simulink model "MechSubTest"  (R2016b)
settings: Solver=VariableStepAuto  StartTime=0.0  StopTime=10.0  RelTol=1e-3
libraries: simulink x1
settings Model: Creator=liana  LastModifiedBy=liana

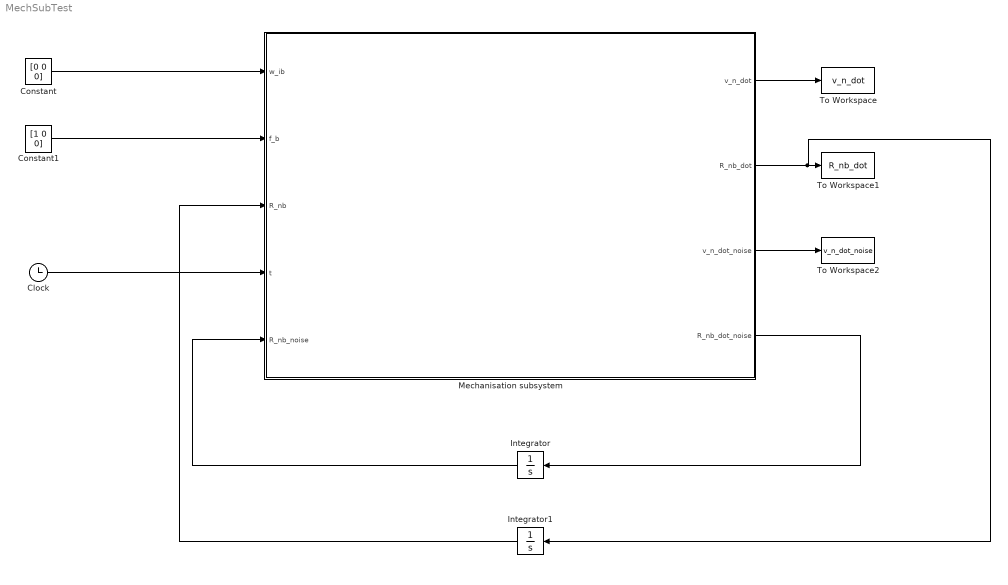
== system MechSubTest ==
  Clock : Clock
  Constant : Constant  Value=[0 0 0]
  Constant1 : Constant  Value=[1 0 0]
  Integrator : Integrator
  Integrator1 : Integrator
  Mechanisation subsystem : Subsystem
  To Workspace : ToWorkspace  VariableName=v_n_dot  SampleTime=-1
  To Workspace1 : ToWorkspace  VariableName=R_nb_dot  SampleTime=-1
  To Workspace2 : ToWorkspace  VariableName=v_n_dot_noise  SampleTime=-1
  wires:
  Constant/1 -> Mechanisation subsystem/1(w_ib)
  Constant1/1 -> Mechanisation subsystem/2(f_b)
  Mechanisation subsystem/2(R_nb_dot) -> Integrator1/1, To Workspace1/1
  Clock/1 -> Mechanisation subsystem/4(t)
  Mechanisation subsystem/4(R_nb_dot_noise) -> Integrator/1
  Integrator/1 -> Mechanisation subsystem/5(R_nb_noise)
  Mechanisation subsystem/1(v_n_dot) -> To Workspace/1
  Mechanisation subsystem/3(v_n_dot_noise) -> To Workspace2/1
  Integrator1/1 -> Mechanisation subsystem/3(R_nb)

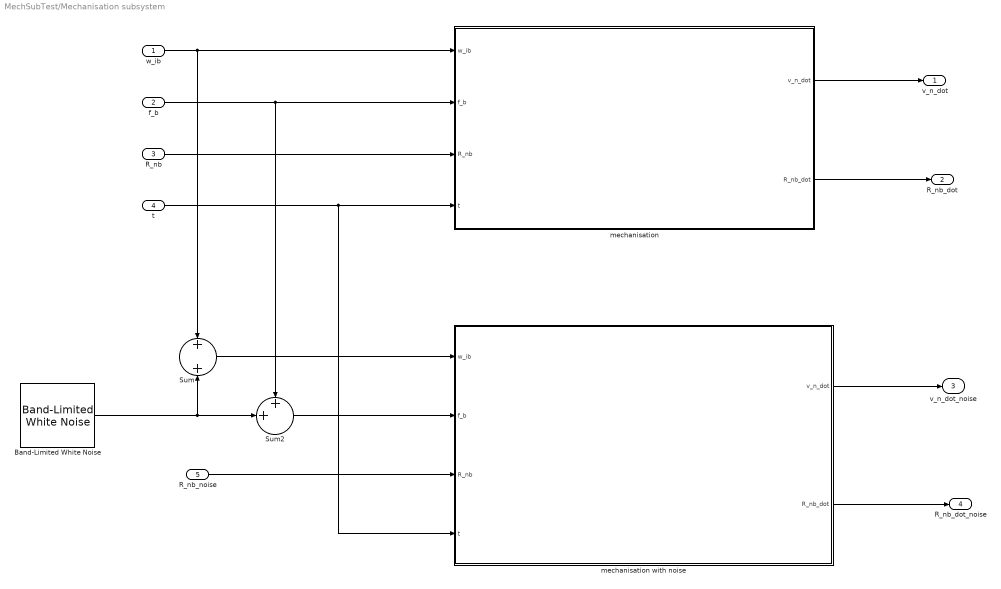
== system MechSubTest/Mechanisation subsystem ==
  w_ib : Inport
  f_b : Inport  Port=2
  R_nb : Inport  Port=3
  t : Inport  Port=4
  R_nb_noise : Inport  Port=5
  Band-Limited White Noise : simulink/Sources/Band-Limited White Noise  Cov=[100 100 100]'  Ts=0.1  seed=[23341]  VectorParams1D=off
  Sum : Sum  Inputs=+|+
  Sum2 : Sum  Inputs=++|
  mechanisation : MATLAB Function  TreatAsAtomicUnit=on
  mechanisation with noise : MATLAB Function  TreatAsAtomicUnit=on
  v_n_dot : Outport
  R_nb_dot : Outport  Port=2
  v_n_dot_noise : Outport  Port=3
  R_nb_dot_noise : Outport  Port=4
  wires:
  w_ib/1 -> mechanisation/1(w_ib), Sum/1
  t/1 -> mechanisation with noise/4(t), mechanisation/4(t)
  R_nb/1 -> mechanisation/3(R_nb)
  f_b/1 -> Sum2/1, mechanisation/2(f_b)
  mechanisation/1(v_n_dot) -> v_n_dot/1
  mechanisation/2(R_nb_dot) -> R_nb_dot/1
  Band-Limited White Noise/1 -> Sum/2, Sum2/2
  Sum/1 -> mechanisation with noise/1(w_ib)
  Sum2/1 -> mechanisation with noise/2(f_b)
  mechanisation with noise/1(v_n_dot) -> v_n_dot_noise/1
  mechanisation with noise/2(R_nb_dot) -> R_nb_dot_noise/1
  R_nb_noise/1 -> mechanisation with noise/3(R_nb)

== matlab function MechSubTest/Mechanisation subsystem/mechanisation ==
  data: w_ib input; f_b input; v_n_dot output; R_nb_dot output; R_nb input; t input
function [v_n_dot, R_nb_dot] = mechanisation(w_ib, f_b, R_nb, t)



g_n = [0 0 9.81]';

% w_ib = size(3,1);

if t == 0
    v_n_dot = zeros(3,1);
    R_nb_dot = eye(3);
    R_nb = eye(3);
end

% mechanisation

% Skew = zeros(3,3);
% Skew(1,2) = -w_ib(3);
% Skew(2,1) = w_ib(3);
% Skew(1,3) = w_ib(2);
% Skew(3,1) = -w_ib(2);
% Skew(2,3) = -w_ib(1);
% Skew(3,2) = w_ib(1);

Skew = skew(w_ib);


%p_dot = v_n;
v_n_dot = R_nb * f_b + g_n;
R_nb_dot = R_nb * Skew;

end

== matlab function MechSubTest/Mechanisation subsystem/mechanisation with noise ==
  data: w_ib input; f_b input; v_n_dot output; R_nb_dot output; R_nb input; t input
function [v_n_dot, R_nb_dot] = mechanisation(w_ib, f_b, R_nb, t)



g_n = [0 0 1]';

% w_ib = size(3,1);

if t == 0
    v_n_dot = zeros(3,1);
    R_nb_dot = eye(3);
    R_nb = eye(3);
end

% mechanisation

% Skew = zeros(3,3);
% Skew(1,2) = -w_ib(3);
% Skew(2,1) = w_ib(3);
% Skew(1,3) = w_ib(2);
% Skew(3,1) = -w_ib(2);
% Skew(2,3) = -w_ib(1);
% Skew(3,2) = w_ib(1);
Skew = skew(w_ib);


%p_dot = v_n;
v_n_dot = R_nb * f_b + g_n;
R_nb_dot = R_nb * Skew;
